simulink model "DeployableEMF"  (R2024a)
settings: Solver=FixedStepAuto  StartTime=0.0  StopTime=0  FixedStep=framePeriod_s  RelTol=1e-3
undefined symbols (not defined in the file): Aircraft, aircraftIC, AircraftModel, Avphi, DiscIntNeverNeededParam, EMF, EnableFF, EnableInputNoise, EnableRCHH, EnableSpeedHold, framePeriod_s, InitCond, Lv, Yv
libraries: simulink x14, simulink_extras x5
(part 2 of 2)

== system DeployableEMF/EMF CLAWS/ACAH EMF1/OnGroundController ==
  cmdsACT : Inport
  Get ACAH Commands1 : Subsystem
      settings: PortSchema="{\"entries\":[{\"content\":{\"sides\":[{\"content\":{\"connectorIds\":[\"In1\"]},\"type\":\"ConnectorPlacement.EquallySpacedRectSide\",\"uuid\":\"7c65b894-e97e-426b-b3a6-5e2b2b7aa780\"},{\"content\":{\"connectorIds\":[\"Out1\"],\"side\":\"RIGHT\"},\"type\":\"ConnectorPlacement.EquallySpacedRectSide\",\"uuid\":\"da5e6856-a2cd-4302-9f49-e9c1cc422564\"},{\"content\":{\"connectorIds\":[\"Out2\"],\"side\":\"TOP\"},\"type\":\"ConnectorPlacement.EquallySpacedRectSide\",\"uuid\":\"a744aea1-4523-47bd-90bf-604bddb972da\"}]},\"type\":\"ConnectorPlacement.EquallySpacedConnector\",\"uuid\":\"254b2f3c-23c2-4cd5-a42e-cd931c0875f5\"}],\"packageUris\":[\"http://schema.mathworks.com/mf0/Connector/R2020b\"],\"version\":\"1.0\"}"
  OL rotor speeds from throttle : Subsystem  Commented=through
  TrimOmegas_OL : Outport
  CmdMoments_Ground : Outport  Port=2
  wires:
  cmdsACT/1 -> Get ACAH Commands1/1(StickInputs)
  Get ACAH Commands1/1(cmdsACAH) -> CmdMoments_Ground/1
  Get ACAH Commands1/2(throttleOmega) -> OL rotor speeds from throttle/1(throttleOmega)
  OL rotor speeds from throttle/1(Omegas_rps) -> TrimOmegas_OL/1

== system DeployableEMF/EMF CLAWS/ACAH EMF1/Rate Saturation ==
  dlat : Inport
  dlon : Inport  Port=2
  dcol : Inport  Port=3
  dped : Inport  Port=4
  Compare To Constant1 : simulink/Logic and Bit Operations/Compare To Constant  relop=<  const=-EMF.MaxCmd.qdot  OutDataTypeStr=boolean
  Compare To Constant2 : simulink/Logic and Bit Operations/Compare To Constant  relop=>  const=EMF.MaxCmd.qdot  OutDataTypeStr=boolean
  Compare To Constant3 : simulink/Logic and Bit Operations/Compare To Constant  relop=<  const=-EMF.MaxCmd.wdot  OutDataTypeStr=boolean
  Compare To Constant4 : simulink/Logic and Bit Operations/Compare To Constant  relop=>  const=EMF.MaxCmd.wdot  OutDataTypeStr=boolean
  Compare To Constant5 : simulink/Logic and Bit Operations/Compare To Constant  relop=<  const=-EMF.MaxCmd.rdot  OutDataTypeStr=boolean
  Compare To Constant6 : simulink/Logic and Bit Operations/Compare To Constant  relop=>  const=EMF.MaxCmd.rdot  OutDataTypeStr=boolean
  Compare To Constant7 : simulink/Logic and Bit Operations/Compare To Constant  relop=<  const=-EMF.MaxCmd.pdot  OutDataTypeStr=boolean
  Compare To Constant8 : simulink/Logic and Bit Operations/Compare To Constant  relop=>  const=EMF.MaxCmd.pdot  OutDataTypeStr=boolean
  Logical Operator{1..4} (4 alike) : Logic  Operator=OR  AllPortsSameDT=off  OutDataTypeStr=boolean
  Mux : Mux
  Saturation : Saturate  UpperLimit=EMF.MaxCmd.pdot  LowerLimit=-EMF.MaxCmd.pdot
  Saturation1 : Saturate  UpperLimit=EMF.MaxCmd.qdot  LowerLimit=-EMF.MaxCmd.qdot
  Saturation2 : Saturate  UpperLimit=EMF.MaxCmd.wdot  LowerLimit=-EMF.MaxCmd.wdot
  Saturation3 : Saturate  UpperLimit=EMF.MaxCmd.rdot  LowerLimit=-EMF.MaxCmd.rdot
  dcol sat : Outport
  dlat sat : Outport  Port=2
  dlon sat : Outport  Port=3
  dped sat : Outport  Port=4
  Flag : Outport  Port=5
  wires:
  Saturation3/1 -> dped sat/1
  Saturation1/1 -> dlon sat/1
  Saturation/1 -> dlat sat/1
  dlat/1 -> Compare To Constant8/1, Compare To Constant7/1, Saturation/1
  Saturation2/1 -> dcol sat/1
  Compare To Constant7/1 -> Logical Operator4/2
  Compare To Constant8/1 -> Logical Operator4/1
  Logical Operator4/1 -> Mux/1
  Logical Operator1/1 -> Mux/2
  Compare To Constant2/1 -> Logical Operator1/1
  Compare To Constant1/1 -> Logical Operator1/2
  dlon/1 -> Compare To Constant2/1, Compare To Constant1/1, Saturation1/1
  dcol/1 -> Compare To Constant3/1, Compare To Constant4/1, Saturation2/1
  Compare To Constant3/1 -> Logical Operator2/2
  Compare To Constant4/1 -> Logical Operator2/1
  Logical Operator2/1 -> Mux/3
  Logical Operator3/1 -> Mux/4
  Compare To Constant6/1 -> Logical Operator3/1
  Compare To Constant5/1 -> Logical Operator3/2
  dped/1 -> Saturation3/1, Compare To Constant6/1, Compare To Constant5/1
  Mux/1 -> Flag/1

== system DeployableEMF/EMF CLAWS/ACAH EMF1/Remap Rotor Speeds to PWM ==
  Rotor Speeds : Inport
  Band-Limited White Noise : simulink/Sources/Band-Limited White Noise  Cov=[1 1 1 1]*0.05  Ts=0.01  seed=[23341 34452 45563 56674]
  Constant1 : Constant  Value=AircraftModel.MinOmegaLimit
  Constant2 : Constant  Value=AircraftModel.MaxOmegaLimit
  Constant3 : Constant  Value=AircraftModel.MinPWMLimit*ones(1,4)
  Constant4 : Constant  Value=AircraftModel.MaxPWMLimit*ones(4,1)
  Data Type Conversion : DataTypeConversion  OutDataTypeStr=int16  SaturateOnIntegerOverflow=off  RndMeth=Floor
  Gain : Gain  Gain=EnableInputNoise
  Rotor Speed Saturation : Subsystem
  Sum1 : Sum  Inputs=|++
  remap : MATLAB Function  TreatAsAtomicUnit=on
  PWM_int16 : Outport
  tag scope: OmSatFlag=global
  wires:
  Sum1/1 -> Data Type Conversion/1  "PWM_cont"
  Rotor Speed Saturation/2(Saturated Rotor Speeds) -> remap/1(norm_in)
  Band-Limited White Noise/1 -> Gain/1
  Rotor Speed Saturation/1(OmegaSaturationFlags) -> [OmSatFlag]
  Data Type Conversion/1 -> PWM_int16/1  "PWM_int16"
  Constant2/1 -> remap/3(in_max)
  remap/1(raw_out) -> Sum1/1  "PWM_cont"
  Constant4/1 -> remap/5(out_max)
  Gain/1 -> Sum1/2
  Constant1/1 -> remap/2(in_min)
  Constant3/1 -> remap/4(out_min)
  Rotor Speeds/1 -> Rotor Speed Saturation/1(Rotor Speeds)

== system DeployableEMF/EMF CLAWS/ACAH EMF1/Subsystem ==
  StateBus : Inport
  Add : Sum  Inputs=+++
  Bus Selector1 : BusSelector  OutputSignals=u_fdbk_mps,v_fdbk_mps,w_fdbk_mps
  Gain : Gain  Gain=0
  Sqrt : Sqrt
  Square : Math  Operator=square
  Square1 : Math  Operator=square
  Square2 : Math  Operator=square
  fps_to_kts : Gain  Gain=0.592484
  Vabs_kts : Outport
  wires:
  Square1/1 -> Add/2
  Bus Selector1/3 -> Square2/1  "<w_fdbk_mps>"
  StateBus/1 -> Bus Selector1/1
  Add/1 -> Sqrt/1
  Square/1 -> Add/1
  Bus Selector1/1 -> Square/1  "<u_fdbk_mps>"
  Bus Selector1/2 -> Gain/1  "<v_fdbk_mps>"
  Sqrt/1 -> fps_to_kts/1
  Square2/1 -> Add/3
  Gain/1 -> Square1/1
  fps_to_kts/1 -> Vabs_kts/1

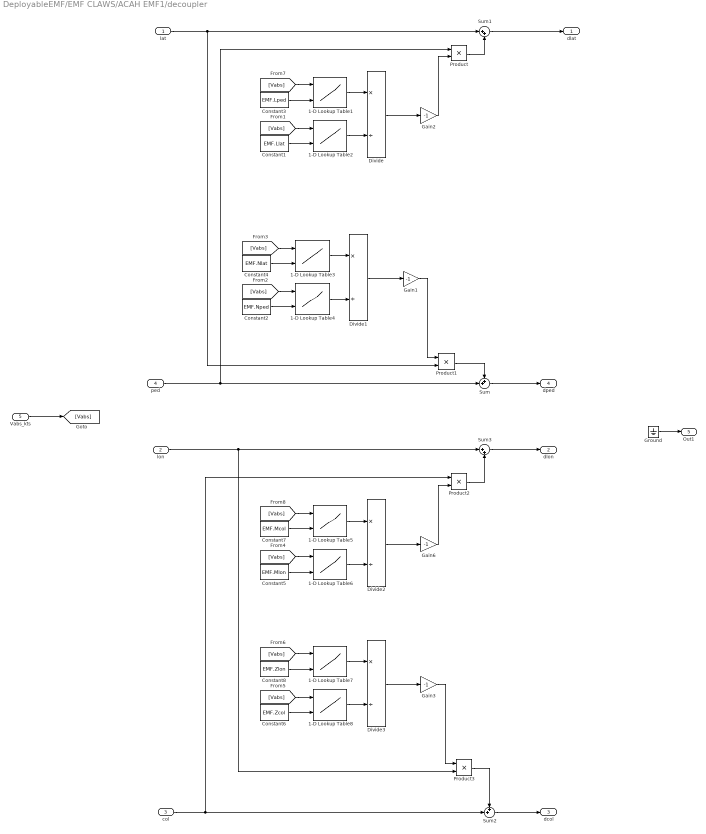
== system DeployableEMF/EMF CLAWS/ACAH EMF1/decoupler ==
  lat : Inport
  lon : Inport  Port=2
  col : Inport  Port=3
  ped : Inport  Port=4
  Vabs_kts : Inport  Port=5
  1-D Lookup Table{1..8} (8 alike) : Lookup_n-D  NumberOfTableDimensions=1  BreakpointsForDimension1=EMF.VTAB  BeginIndexSearchUsingPreviousIndexResult=on  TableSource=Input port  Table=tanh([-5:5])  ExtrapMethod=Clip  InternalRulePriority=Speed  RndMeth=Simplest
      settings: InputPortMap=u0,p221
  Constant1 : Constant  Value=EMF.Llat
  Constant2 : Constant  Value=EMF.Nped
  Constant3 : Constant  Value=EMF.Lped
  Constant4 : Constant  Value=EMF.Nlat
  Constant5 : Constant  Value=EMF.Mlon
  Constant6 : Constant  Value=EMF.Zcol
  Constant7 : Constant  Value=EMF.Mcol
  Constant8 : Constant  Value=EMF.Zlon
  Divide{,1..3} (4 alike) : Product  Inputs=*/
  Gain{1..3,6} (4 alike) : Gain  Gain=-1
  Ground : Ground
  Product{,1..3} (4 alike) : Product
  Sum : Sum  Inputs=++|
  Sum1 : Sum  Inputs=|++
  Sum2 : Sum  Inputs=++|
  Sum3 : Sum  Inputs=|++
  dlat : Outport
  dlon : Outport  Port=2
  dcol : Outport  Port=3
  dped : Outport  Port=4
  Out1 : Outport  Port=5
  wires:
  Vabs_kts/1 -> [Vabs]
  Product3/1 -> Sum2/1
  Product2/1 -> Sum3/2
  Constant7/1 -> 1-D Lookup Table5/2
  [Vabs] -> 1-D Lookup Table5/1
  [Vabs] -> 1-D Lookup Table6/1
  Constant5/1 -> 1-D Lookup Table6/2
  1-D Lookup Table6/1 -> Divide2/2
  1-D Lookup Table5/1 -> Divide2/1
  Divide2/1 -> Gain6/1
  Gain6/1 -> Product2/2
  Gain3/1 -> Product3/1
  Divide3/1 -> Gain3/1
  1-D Lookup Table7/1 -> Divide3/1
  1-D Lookup Table8/1 -> Divide3/2
  Constant6/1 -> 1-D Lookup Table8/2
  [Vabs] -> 1-D Lookup Table8/1
  [Vabs] -> 1-D Lookup Table7/1
  Constant8/1 -> 1-D Lookup Table7/2
  Product1/1 -> Sum/1
  Constant4/1 -> 1-D Lookup Table3/2
  [Vabs] -> 1-D Lookup Table3/1
  [Vabs] -> 1-D Lookup Table4/1
  Constant2/1 -> 1-D Lookup Table4/2
  1-D Lookup Table4/1 -> Divide1/2
  1-D Lookup Table3/1 -> Divide1/1
  Divide1/1 -> Gain1/1
  Gain1/1 -> Product1/1
  Gain2/1 -> Product/2
  Product/1 -> Sum1/2
  Divide/1 -> Gain2/1
  1-D Lookup Table1/1 -> Divide/1
  1-D Lookup Table2/1 -> Divide/2
  Constant1/1 -> 1-D Lookup Table2/2
  [Vabs] -> 1-D Lookup Table2/1
  [Vabs] -> 1-D Lookup Table1/1
  Constant3/1 -> 1-D Lookup Table1/2
  Sum3/1 -> dlon/1
  Sum2/1 -> dcol/1
  Sum1/1 -> dlat/1
  ped/1 -> Sum/2, Product/1
  lat/1 -> Sum1/1, Product1/2
  Sum/1 -> dped/1
  col/1 -> Product2/1, Sum2/2
  lon/1 -> Product3/2, Sum3/1
  Ground/1 -> Out1/1

== system DeployableEMF/EMF CLAWS/ACAH EMF1/Inner Loop - ACAH/A-channel Delay ==
  p_ideal : Inport
  phi_ideal : Inport  Port=2
  Constant : Constant  Value=EMF.tauf
  Demux : Demux  Outputs=2
  Divide : Product  Inputs=*/
  Integrator : Integrator
  Mux : Mux  Inputs=2
  Sum : Sum  Inputs=|+-
  p_ideal_delayed : Outport
  phi_ideal_delayed : Outport  Port=2
  wires:
  Demux/2 -> phi_ideal_delayed/1
  Demux/1 -> p_ideal_delayed/1
  phi_ideal/1 -> Mux/2
  p_ideal/1 -> Mux/1
  Mux/1 -> Sum/1
  Constant/1 -> Divide/2
  Divide/1 -> Integrator/1
  Sum/1 -> Divide/1
  Integrator/1 -> Demux/1, Sum/2

== system DeployableEMF/EMF CLAWS/ACAH EMF1/Inner Loop - ACAH/B-channel Delay ==
  q_ideal : Inport
  tht_ideal : Inport  Port=2
  Constant : Constant  Value=EMF.tauf
  Demux : Demux  Outputs=2
  Divide : Product  Inputs=*/
  Integrator : Integrator
  Mux : Mux  Inputs=2
  Sum : Sum  Inputs=|+-
  q_ideal_delayed : Outport
  tht_ideal_delayed : Outport  Port=2
  wires:
  Demux/2 -> tht_ideal_delayed/1
  Demux/1 -> q_ideal_delayed/1
  tht_ideal/1 -> Mux/2
  q_ideal/1 -> Mux/1
  Mux/1 -> Sum/1
  Constant/1 -> Divide/2
  Divide/1 -> Integrator/1
  Sum/1 -> Divide/1
  Integrator/1 -> Demux/1, Sum/2

== system DeployableEMF/EMF CLAWS/ACAH EMF1/Inner Loop - ACAH/C-channel Delay ==
  w_ideal : Inport
  Constant : Constant  Value=EMF.tauf
  Divide : Product  Inputs=*/
  Integrator : Integrator
  Sum : Sum  Inputs=|+-
  w_ideal_delay : Outport
  wires:
  w_ideal/1 -> Sum/1
  Constant/1 -> Divide/2
  Divide/1 -> Integrator/1
  Sum/1 -> Divide/1
  Integrator/1 -> w_ideal_delay/1, Sum/2

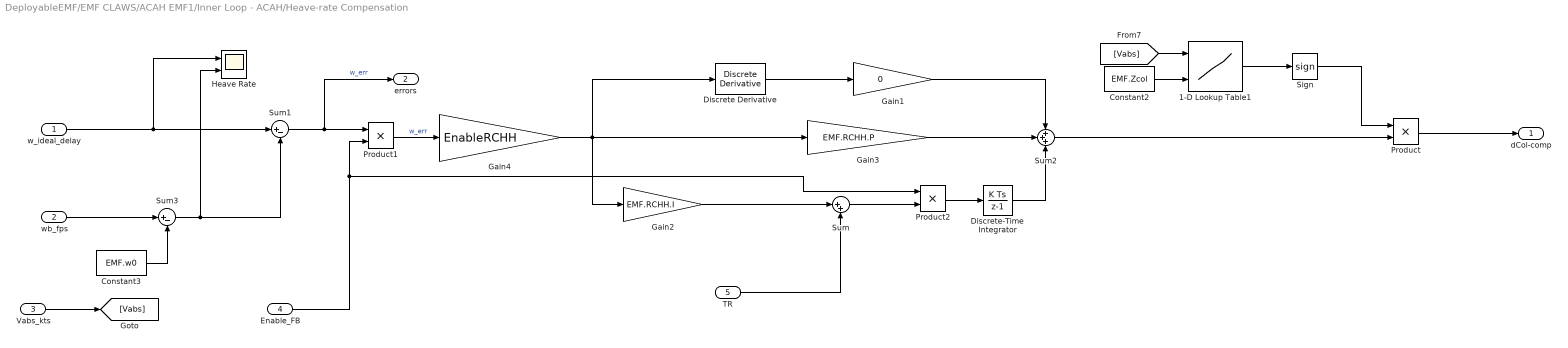
== system DeployableEMF/EMF CLAWS/ACAH EMF1/Inner Loop - ACAH/Heave-rate Compensation ==
  w_ideal_delay : Inport
  wb_fps : Inport  Port=2
  Vabs_kts : Inport  Port=3
  Enable_FB : Inport  Port=4
  TR : Inport  Port=5
  1-D Lookup Table1 : Lookup_n-D  NumberOfTableDimensions=1  BreakpointsForDimension1=EMF.VTAB  BeginIndexSearchUsingPreviousIndexResult=on  TableSource=Input port  Table=tanh([-5:5])  ExtrapMethod=Clip  InternalRulePriority=Speed  RndMeth=Simplest
      settings: InputPortMap=u0,p221
  Constant2 : Constant  Value=EMF.Zcol
  Constant3 : Constant  Value=EMF.w0
  Discrete Derivative : simulink/Discrete/Discrete Derivative  gainval=1.0  ICPrevScaledInput=0.0  OutMin=[]  OutMax=[]  OutDataType=fixdt(1, 16)  OutScaling=2^-10  DoSatur=off
  Discrete-Time Integrator : DiscreteIntegrator  SampleTime=-1  ICPrevOutput=DiscIntNeverNeededParam  ICPrevScaledInput=DiscIntNeverNeededParam
  Gain1 : Gain  Gain=0
  Gain2 : Gain  Gain=EMF.RCHH.I
  Gain3 : Gain  Gain=EMF.RCHH.P
  Gain4 : Gain  Gain=EnableRCHH
  Heave Rate : Scope  NumInputPorts=2
  Product : Product
  Product1 : Product
  Product2 : Product
  Sign : Signum
  Sum : Sum  Inputs=|++
  Sum1 : Sum  Inputs=|+-
  Sum2 : Sum  Inputs=+++
  Sum3 : Sum  Inputs=|+-
  dCol-comp : Outport
  errors : Outport  Port=2
  wires:
  Gain3/1 -> Sum2/2
  Sum/1 -> Product2/2
  wb_fps/1 -> Sum3/1
  Sign/1 -> Product/1
  1-D Lookup Table1/1 -> Sign/1
  Product/1 -> dCol-comp/1
  Discrete Derivative/1 -> Gain1/1
  Product1/1 -> Gain4/1  "w_err"
  Sum2/1 -> Product/2
  Gain1/1 -> Sum2/1
  w_ideal_delay/1 -> Heave Rate/1, Sum1/1
  [Vabs] -> 1-D Lookup Table1/1
  Constant2/1 -> 1-D Lookup Table1/2
  Vabs_kts/1 -> [Vabs]
  Sum3/1 -> Heave Rate/2, Sum1/2
  Constant3/1 -> Sum3/2
  Sum1/1 -> errors/1, Product1/1  "w_err"
  Enable_FB/1 -> Product2/1, Product1/2
  Discrete-Time Integrator/1 -> Sum2/3
  Product2/1 -> Discrete-Time Integrator/1
  Gain2/1 -> Sum/1
  TR/1 -> Sum/2
  Gain4/1 -> Discrete Derivative/1, Gain3/1, Gain2/1

== system DeployableEMF/EMF CLAWS/ACAH EMF1/Inner Loop - ACAH/P-channel Delay ==
  r_ideal : Inport
  Constant : Constant  Value=EMF.tauf
  Divide : Product  Inputs=*/
  Integrator : Integrator
  Sum : Sum  Inputs=|+-
  r_ideal_delay : Outport
  wires:
  Divide/1 -> Integrator/1
  r_ideal/1 -> Sum/1
  Integrator/1 -> Sum/2, r_ideal_delay/1
  Constant/1 -> Divide/2
  Sum/1 -> Divide/1

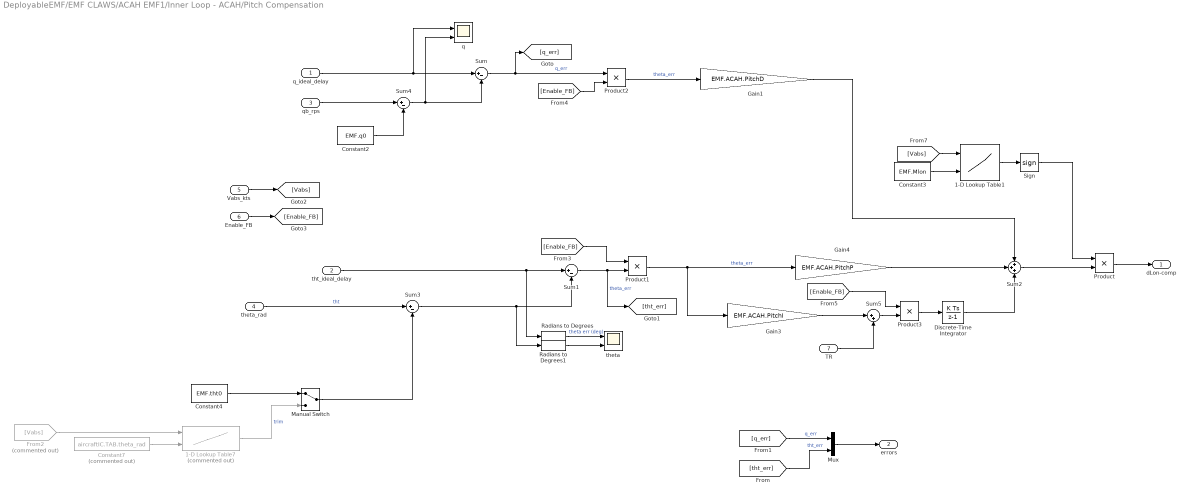
== system DeployableEMF/EMF CLAWS/ACAH EMF1/Inner Loop - ACAH/Pitch Compensation ==
  q_ideal_delay : Inport
  tht_ideal_delay : Inport  Port=2
  qb_rps : Inport  Port=3
  theta_rad : Inport  Port=4
  Vabs_kts : Inport  Port=5
  Enable_FB : Inport  Port=6
  TR : Inport  Port=7
  1-D Lookup Table1 : Lookup_n-D  NumberOfTableDimensions=1  BreakpointsForDimension1=EMF.VTAB  BeginIndexSearchUsingPreviousIndexResult=on  TableSource=Input port  Table=tanh([-5:5])  ExtrapMethod=Clip  InternalRulePriority=Speed  RndMeth=Simplest
      settings: InputPortMap=u0,p221
  1-D Lookup Table7 : Lookup_n-D  Commented=on  NumberOfTableDimensions=1  BreakpointsForDimension1=EMF.VTAB  BeginIndexSearchUsingPreviousIndexResult=on  TableSource=Input port  Table=tanh([-5:5])  ExtrapMethod=Clip  InternalRulePriority=Speed  RndMeth=Simplest
      settings: InputPortMap=u0,p221
  Constant2 : Constant  Value=EMF.q0
  Constant3 : Constant  Value=EMF.Mlon
  Constant4 : Constant  Value=EMF.tht0
  Constant7 : Constant  Commented=on  Value=aircraftIC.TAB.theta_rad
  Discrete-Time Integrator : DiscreteIntegrator  SampleTime=-1  ICPrevOutput=DiscIntNeverNeededParam  ICPrevScaledInput=DiscIntNeverNeededParam
  From2 : From  Commented=on  GotoTag=Vabs
  Gain1 : Gain  Gain=EMF.ACAH.PitchD
  Gain3 : Gain  Gain=EMF.ACAH.PitchI
  Gain4 : Gain  Gain=EMF.ACAH.PitchP
  Manual Switch : ManualSwitch
  Mux : Mux  Inputs=2
  Product{,1..3} (4 alike) : Product
  Radians to Degrees : simulink_extras/Transformations/Radians to Degrees
  Radians to Degrees1 : simulink_extras/Transformations/Radians to Degrees
  Sign : Signum
  Sum{,1,3..4} (4 alike) : Sum  Inputs=|+-
  Sum2 : Sum  Inputs=+++
  Sum5 : Sum  Inputs=|++
  q : Scope  NumInputPorts=2
  theta : Scope  NumInputPorts=2
  dLon-comp : Outport
  errors : Outport  Port=2
  wires:
  Gain4/1 -> Sum2/2
  Sign/1 -> Product/1
  Product/1 -> dLon-comp/1
  Gain1/1 -> Sum2/1
  [q_err] -> Mux/1  "q_err"
  Mux/1 -> errors/1
  [tht_err] -> Mux/2  "tht_err"
  Sum/1 -> Product2/1, [q_err]  "q_err"
  Product1/1 -> Gain3/1, Gain4/1  "theta_err"
  q_ideal_delay/1 -> Sum/1, q/1
  qb_rps/1 -> Sum4/1
  Sum4/1 -> Sum/2, q/2
  Constant2/1 -> Sum4/2
  [Vabs] -> 1-D Lookup Table1/1
  Constant3/1 -> 1-D Lookup Table1/2
  1-D Lookup Table1/1 -> Sign/1
  Vabs_kts/1 -> [Vabs]
  Radians to Degrees/1 -> theta/1  "theta err (deg)"
  Radians to Degrees1/1 -> theta/2
  Constant7/1 -> 1-D Lookup Table7/2
  Constant4/1 -> Manual Switch/1
  Sum3/1 -> Sum1/2, Radians to Degrees1/1
  From2/1 -> 1-D Lookup Table7/1
  theta_rad/1 -> Sum3/1  "tht"
  1-D Lookup Table7/1 -> Manual Switch/2  "trim"
  Sum5/1 -> Product3/2
  tht_ideal_delay/1 -> Sum1/1, Radians to Degrees/1
  Sum2/1 -> Product/2
  Manual Switch/1 -> Sum3/2
  Sum1/1 -> [tht_err], Product1/2  "theta_err"
  Enable_FB/1 -> [Enable_FB]
  [Enable_FB] -> Product1/1
  Product2/1 -> Gain1/1  "theta_err"
  [Enable_FB] -> Product2/2
  Discrete-Time Integrator/1 -> Sum2/3
  Product3/1 -> Discrete-Time Integrator/1
  [Enable_FB] -> Product3/1
  Gain3/1 -> Sum5/1
  TR/1 -> Sum5/2

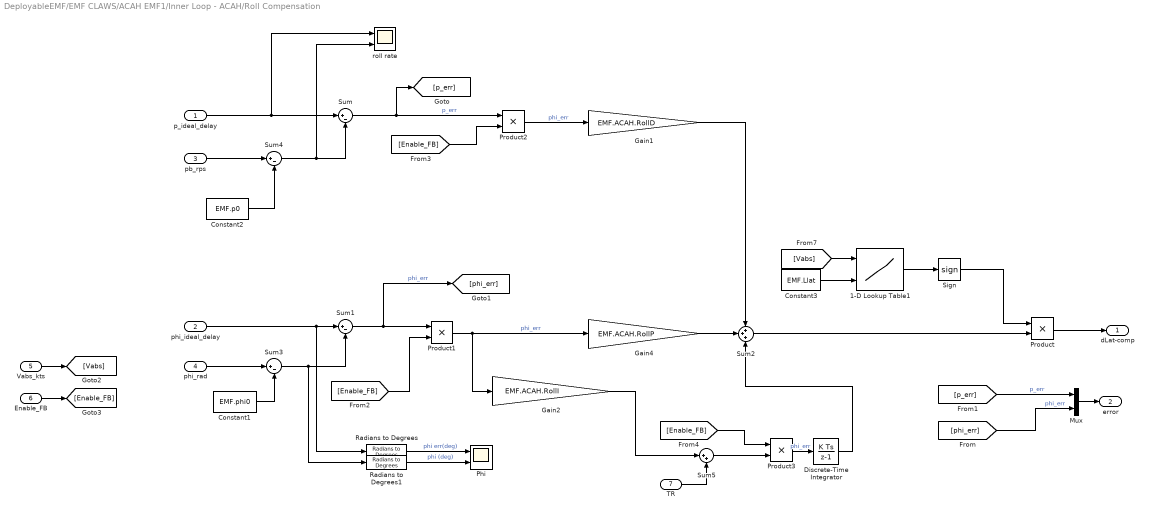
== system DeployableEMF/EMF CLAWS/ACAH EMF1/Inner Loop - ACAH/Roll Compensation ==
  p_ideal_delay : Inport
  phi_ideal_delay : Inport  Port=2
  pb_rps : Inport  Port=3
  phi_rad : Inport  Port=4
  Vabs_kts : Inport  Port=5
  Enable_FB : Inport  Port=6
  TR : Inport  Port=7
  1-D Lookup Table1 : Lookup_n-D  NumberOfTableDimensions=1  BreakpointsForDimension1=EMF.VTAB  BeginIndexSearchUsingPreviousIndexResult=on  TableSource=Input port  Table=tanh([-5:5])  ExtrapMethod=Clip  InternalRulePriority=Speed  RndMeth=Simplest
      settings: InputPortMap=u0,p221
  Constant1 : Constant  Value=EMF.phi0
  Constant2 : Constant  Value=EMF.p0
  Constant3 : Constant  Value=EMF.Llat
  Discrete-Time Integrator : DiscreteIntegrator  SampleTime=-1  ICPrevOutput=DiscIntNeverNeededParam  ICPrevScaledInput=DiscIntNeverNeededParam
  Gain1 : Gain  Gain=EMF.ACAH.RollD
  Gain2 : Gain  Gain=EMF.ACAH.RollI
  Gain4 : Gain  Gain=EMF.ACAH.RollP
  Mux : Mux  Inputs=2
  Phi : Scope  NumInputPorts=2
  Product{,1..3} (4 alike) : Product
  Radians to Degrees : simulink_extras/Transformations/Radians to Degrees
  Radians to Degrees1 : simulink_extras/Transformations/Radians to Degrees
  Sign : Signum
  Sum{,1,3..4} (4 alike) : Sum  Inputs=|+-
  Sum2 : Sum  Inputs=+++
  Sum5 : Sum  Inputs=|++
  roll rate : Scope  NumInputPorts=2
  dLat-comp : Outport
  error : Outport  Port=2
  wires:
  Gain4/1 -> Sum2/2
  Sum2/1 -> Product/2
  Sign/1 -> Product/1
  Product/1 -> dLat-comp/1
  [phi_err] -> Mux/2  "phi_err"
  phi_ideal_delay/1 -> Sum1/1, Radians to Degrees/1
  phi_rad/1 -> Sum3/1
  Sum/1 -> [p_err], Product2/1  "p_err"
  Gain1/1 -> Sum2/1
  Product1/1 -> Gain2/1, Gain4/1  "phi_err"
  p_ideal_delay/1 -> Sum/1, roll rate/1
  Sum3/1 -> Radians to Degrees1/1, Sum1/2
  Constant1/1 -> Sum3/2
  Sum4/1 -> Sum/2, roll rate/2
  Constant2/1 -> Sum4/2
  pb_rps/1 -> Sum4/1
  [Vabs] -> 1-D Lookup Table1/1
  Constant3/1 -> 1-D Lookup Table1/2
  Vabs_kts/1 -> [Vabs]
  1-D Lookup Table1/1 -> Sign/1
  Sum5/1 -> Product3/2
  Radians to Degrees/1 -> Phi/1  "phi err(deg)"
  Radians to Degrees1/1 -> Phi/2  "phi (deg)"
  Enable_FB/1 -> [Enable_FB]
  Sum1/1 -> [phi_err], Product1/1  "phi_err"
  [Enable_FB] -> Product1/2
  Product2/1 -> Gain1/1  "phi_err"
  [Enable_FB] -> Product2/2
  Discrete-Time Integrator/1 -> Sum2/3
  Product3/1 -> Discrete-Time Integrator/1  "phi_err"
  [Enable_FB] -> Product3/1
  Gain2/1 -> Sum5/1
  TR/1 -> Sum5/2
  Mux/1 -> error/1
  [p_err] -> Mux/1  "p_err"

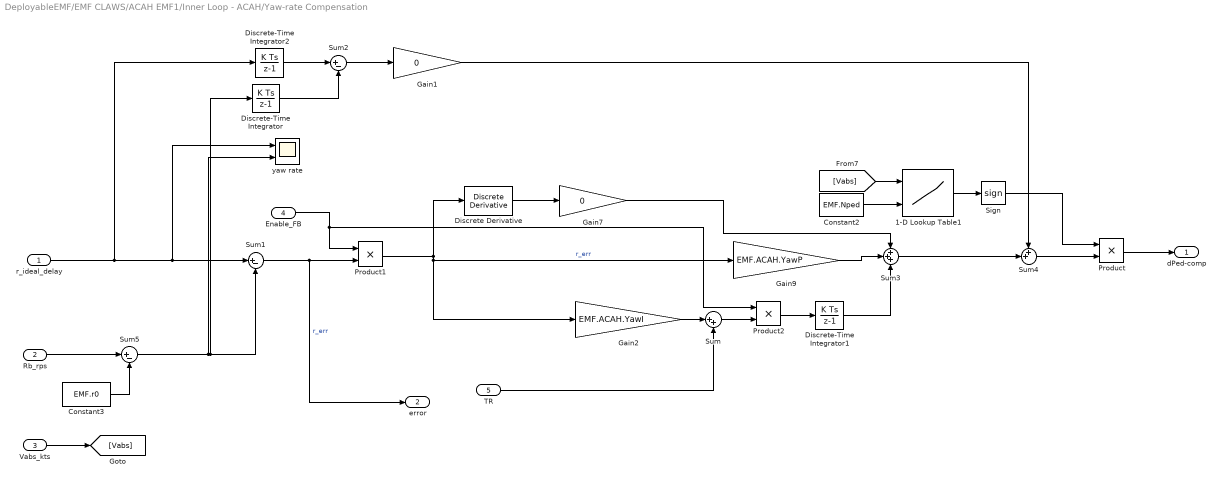
== system DeployableEMF/EMF CLAWS/ACAH EMF1/Inner Loop - ACAH/Yaw-rate Compensation ==
  r_ideal_delay : Inport
  Rb_rps : Inport  Port=2
  Vabs_kts : Inport  Port=3
  Enable_FB : Inport  Port=4
  TR : Inport  Port=5
  1-D Lookup Table1 : Lookup_n-D  NumberOfTableDimensions=1  BreakpointsForDimension1=EMF.VTAB  BeginIndexSearchUsingPreviousIndexResult=on  TableSource=Input port  Table=tanh([-5:5])  ExtrapMethod=Clip  InternalRulePriority=Speed  RndMeth=Simplest
      settings: InputPortMap=u0,p221
  Constant2 : Constant  Value=EMF.Nped
  Constant3 : Constant  Value=EMF.r0
  Discrete Derivative : simulink/Discrete/Discrete Derivative  gainval=1.0  ICPrevScaledInput=0.0  OutMin=[]  OutMax=[]  OutDataType=fixdt(1, 16)  OutScaling=2^-10  DoSatur=off
  Discrete-Time Integrator : DiscreteIntegrator  SampleTime=-1  ICPrevOutput=DiscIntNeverNeededParam  ICPrevScaledInput=DiscIntNeverNeededParam
  Discrete-Time Integrator1 : DiscreteIntegrator  SampleTime=-1  ICPrevOutput=DiscIntNeverNeededParam  ICPrevScaledInput=DiscIntNeverNeededParam
  Discrete-Time Integrator2 : DiscreteIntegrator  SampleTime=-1  ICPrevOutput=DiscIntNeverNeededParam  ICPrevScaledInput=DiscIntNeverNeededParam
  Gain1 : Gain  Gain=0
  Gain2 : Gain  Gain=EMF.ACAH.YawI
  Gain7 : Gain  Gain=0
  Gain9 : Gain  Gain=EMF.ACAH.YawP
  Product : Product
  Product1 : Product
  Product2 : Product
  Sign : Signum
  Sum : Sum  Inputs=|++
  Sum1 : Sum  Inputs=|+-
  Sum2 : Sum  Inputs=|+-
  Sum3 : Sum  Inputs=+++
  Sum4 : Sum  Inputs=++|
  Sum5 : Sum  Inputs=|+-
  yaw rate : Scope  NumInputPorts=2
  dPed-comp : Outport
  error : Outport  Port=2
  wires:
  Product1/1 -> Discrete Derivative/1, Gain2/1, Gain9/1  "r_err"
  Discrete Derivative/1 -> Gain7/1
  Gain7/1 -> Sum3/1
  Gain9/1 -> Sum3/2
  Sum/1 -> Product2/2
  Sign/1 -> Product/1
  Product/1 -> dPed-comp/1
  1-D Lookup Table1/1 -> Sign/1
  Rb_rps/1 -> Sum5/1
  r_ideal_delay/1 -> Discrete-Time Integrator2/1, Sum1/1, yaw rate/1
  Discrete-Time Integrator2/1 -> Sum2/1
  Discrete-Time Integrator/1 -> Sum2/2
  Sum2/1 -> Gain1/1
  Sum3/1 -> Sum4/2
  Sum4/1 -> Product/2
  Gain1/1 -> Sum4/1
  [Vabs] -> 1-D Lookup Table1/1
  Constant2/1 -> 1-D Lookup Table1/2
  Vabs_kts/1 -> [Vabs]
  Sum5/1 -> Discrete-Time Integrator/1, Sum1/2, yaw rate/2
  Constant3/1 -> Sum5/2
  Enable_FB/1 -> Product2/1, Product1/1
  Sum1/1 -> error/1, Product1/2  "r_err"
  Discrete-Time Integrator1/1 -> Sum3/3
  Product2/1 -> Discrete-Time Integrator1/1
  Gain2/1 -> Sum/1
  TR/1 -> Sum/2

== system DeployableEMF/EMF CLAWS/ACAH EMF1/Inner Loop - ACAH/[Heave] Cmd Filter // Inv Model ==
  note: Inverse Model
  note: Command Filter
  w_cmd (ft/s) : Inport
  Vabs_kts : Inport  Port=2
  1-D Lookup Table : Lookup_n-D  NumberOfTableDimensions=1  BreakpointsForDimension1=EMF.VTAB  BeginIndexSearchUsingPreviousIndexResult=on  TableSource=Input port  Table=tanh([-5:5])  ExtrapMethod=Clip  InternalRulePriority=Speed  OutDataTypeStr=single  RndMeth=Simplest
      settings: InputPortMap=u0,p221
  1-D Lookup Table1 : Lookup_n-D  NumberOfTableDimensions=1  BreakpointsForDimension1=EMF.VTAB  BeginIndexSearchUsingPreviousIndexResult=on  TableSource=Input port  Table=tanh([-5:5])  ExtrapMethod=Clip  InternalRulePriority=Speed  OutDataTypeStr=single  RndMeth=Simplest
      settings: InputPortMap=u0,p221
  Bus Creator : BusCreator  Inputs=2
  Constant : Constant  Value=EMF.wTau  OutDataTypeStr=single
  Constant1 : Constant  Value=EMF.Zw  OutDataTypeStr=single
  Constant3 : Constant  Value=EMF.Zcol  OutDataTypeStr=single
  Delay : Delay  DelayLength=EMF.HeaveDelay/framePeriod_s
  Delay1 : Delay  DelayLength=EMF.HeaveDelay/framePeriod_s
  Discrete-Time Integrator : DiscreteIntegrator  SampleTime=-1  OutDataTypeStr=single  ICPrevOutput=DiscIntNeverNeededParam  ICPrevScaledInput=DiscIntNeverNeededParam
  Divide : Product  Inputs=*/  OutDataTypeStr=single
  Divide1 : Product  Inputs=*/  OutDataTypeStr=single
  Product3 : Product
  Sum : Sum  Inputs=|+-
  Sum2 : Sum  Inputs=|+-
  col_ff : Outport
  w_ideal : Outport  Port=2
  cmdFilValues : Outport  Port=3
  wires:
  [wdot_ideal] -> Delay/1  "wdot_ideal"
  [w_ideal] -> Delay1/1  "Vz_ideal"
  Bus Creator/1 -> cmdFilValues/1
  Divide/1 -> Discrete-Time Integrator/1, Sum2/1, [wdot_ideal]  "wdot_ideal"
  Discrete-Time Integrator/1 -> w_ideal/1, [w_ideal], Product3/2, Sum/2  "w_ideal"
  Sum/1 -> Divide/1
  w_cmd (ft/s)/1 -> Sum/1
  Sum2/1 -> Divide1/1
  Constant/1 -> Divide/2
  Product3/1 -> Sum2/2
  Divide1/1 -> col_ff/1
  [Vabs] -> 1-D Lookup Table/1
  Constant1/1 -> 1-D Lookup Table/2
  1-D Lookup Table/1 -> Product3/1
  [Vabs] -> 1-D Lookup Table1/1
  Constant3/1 -> 1-D Lookup Table1/2
  1-D Lookup Table1/1 -> Divide1/2
  Vabs_kts/1 -> [Vabs]
  Delay/1 -> Bus Creator/1  "Vzdot_filtered"
  Delay1/1 -> Bus Creator/2  "Vz_filtered"

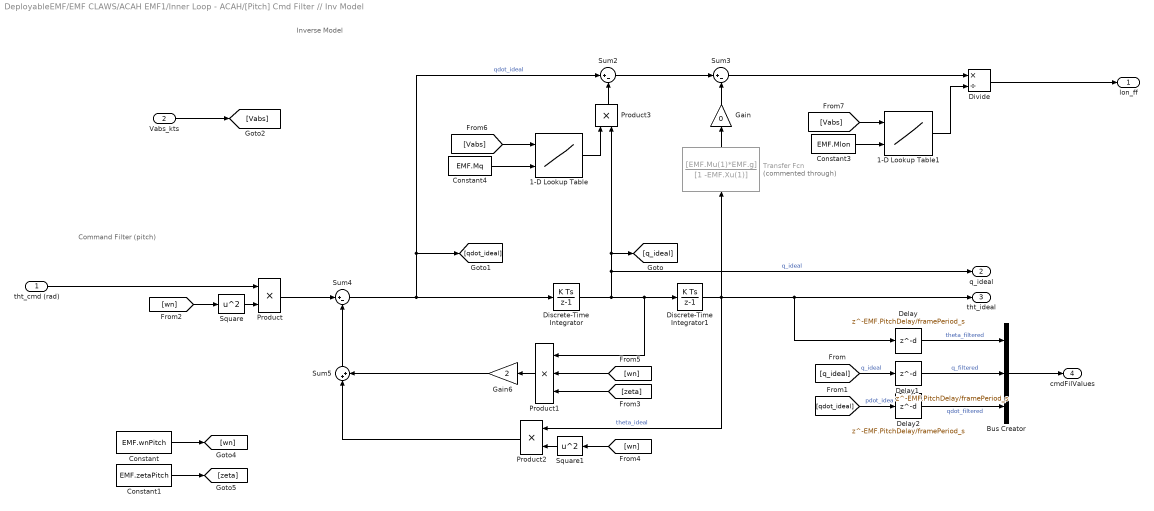
== system DeployableEMF/EMF CLAWS/ACAH EMF1/Inner Loop - ACAH/[Pitch] Cmd Filter // Inv Model ==
  note: Command Filter (pitch)
  note: Inverse Model
  tht_cmd (rad) : Inport
  Vabs_kts : Inport  Port=2
  1-D Lookup Table : Lookup_n-D  NumberOfTableDimensions=1  BreakpointsForDimension1=EMF.VTAB  BeginIndexSearchUsingPreviousIndexResult=on  TableSource=Input port  Table=tanh([-5:5])  ExtrapMethod=Clip  InternalRulePriority=Speed  RndMeth=Simplest
      settings: InputPortMap=u0,p221
  1-D Lookup Table1 : Lookup_n-D  NumberOfTableDimensions=1  BreakpointsForDimension1=EMF.VTAB  BeginIndexSearchUsingPreviousIndexResult=on  TableSource=Input port  Table=tanh([-5:5])  ExtrapMethod=Clip  InternalRulePriority=Speed  RndMeth=Simplest
      settings: InputPortMap=u0,p221
  Bus Creator : BusCreator  Inputs=3
  Constant : Constant  Value=EMF.wnPitch
  Constant1 : Constant  Value=EMF.zetaPitch
  Constant3 : Constant  Value=EMF.Mlon
  Constant4 : Constant  Value=EMF.Mq
  Delay : Delay  DelayLength=EMF.PitchDelay/framePeriod_s
  Delay1 : Delay  DelayLength=EMF.PitchDelay/framePeriod_s
  Delay2 : Delay  DelayLength=EMF.PitchDelay/framePeriod_s
  Discrete-Time Integrator : DiscreteIntegrator  SampleTime=-1  ICPrevOutput=DiscIntNeverNeededParam  ICPrevScaledInput=DiscIntNeverNeededParam
  Discrete-Time Integrator1 : DiscreteIntegrator  SampleTime=-1  ICPrevOutput=DiscIntNeverNeededParam  ICPrevScaledInput=DiscIntNeverNeededParam
  Divide : Product  Inputs=*/
  Gain : Gain  Gain=0
  Gain6 : Gain  Gain=2
  Product : Product
  Product1 : Product  Inputs=3
  Product2 : Product
  Product3 : Product
  Square : Math  Operator=square
  Square1 : Math  Operator=square
  Sum2 : Sum  Inputs=|+-
  Sum3 : Sum  Inputs=|+-
  Sum4 : Sum  Inputs=|+-
  Sum5 : Sum  Inputs=|++
  Transfer Fcn : TransferFcn  Commented=through  Numerator=[EMF.Mu(1)*EMF.g]  Denominator=[1 -EMF.Xu(1)]
  lon_ff : Outport
  q_ideal : Outport  Port=2
  tht_ideal : Outport  Port=3
  cmdFilValues : Outport  Port=4
  wires:
  [q_ideal] -> Delay1/1  "q_ideal"
  [qdot_ideal] -> Delay2/1  "pdot_idea"
  Bus Creator/1 -> cmdFilValues/1
  Sum2/1 -> Sum3/1
  tht_cmd (rad)/1 -> Product/1
  Transfer Fcn/1 -> Gain/1
  [wn] -> Product1/2
  Product1/1 -> Gain6/1
  [zeta] -> Product1/3
  Constant1/1 -> [zeta]
  Gain6/1 -> Sum5/2
  Product/1 -> Sum4/1
  Constant/1 -> [wn]
  Square1/1 -> Product2/2
  [wn] -> Square1/1
  Square/1 -> Product/2
  Discrete-Time Integrator/1 -> Product3/2, [q_ideal], q_ideal/1, Discrete-Time Integrator1/1, Product1/1  "q_ideal"
  [wn] -> Square/1
  Discrete-Time Integrator1/1 -> Delay/1, tht_ideal/1, Transfer Fcn/1, Product2/1  "theta_ideal"
  Sum4/1 -> Discrete-Time Integrator/1, [qdot_ideal], Sum2/1  "qdot_ideal"
  Sum5/1 -> Sum4/2
  Product2/1 -> Sum5/1
  1-D Lookup Table/1 -> Product3/1
  Product3/1 -> Sum2/2
  Sum3/1 -> Divide/1
  Divide/1 -> lon_ff/1
  Gain/1 -> Sum3/2
  [Vabs] -> 1-D Lookup Table/1
  Constant4/1 -> 1-D Lookup Table/2
  Constant3/1 -> 1-D Lookup Table1/2
  1-D Lookup Table1/1 -> Divide/2
  [Vabs] -> 1-D Lookup Table1/1
  Vabs_kts/1 -> [Vabs]
  Delay/1 -> Bus Creator/1  "theta_filtered"
  Delay1/1 -> Bus Creator/2  "q_filtered"
  Delay2/1 -> Bus Creator/3  "qdot_filtered"

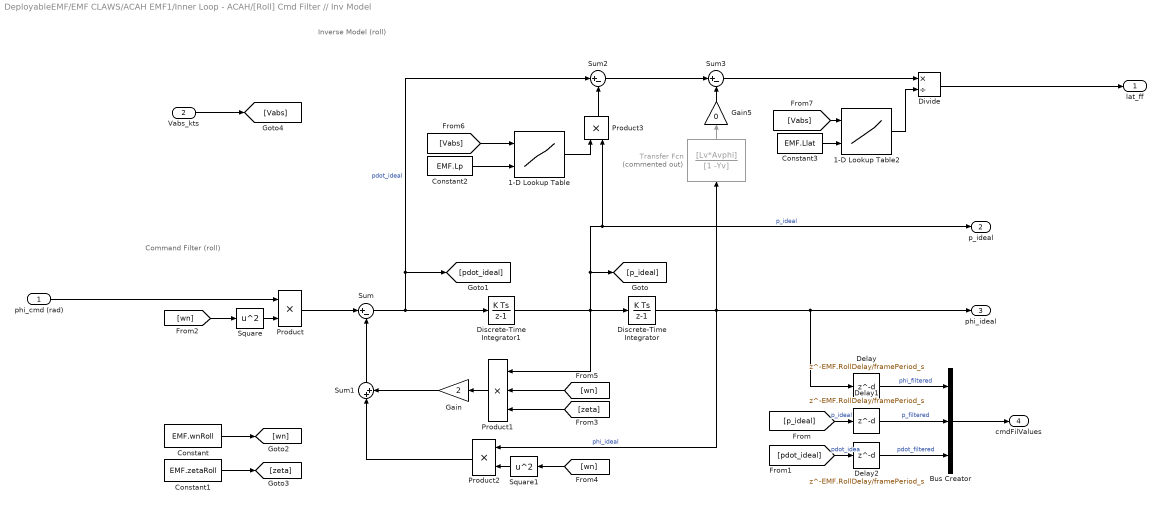
== system DeployableEMF/EMF CLAWS/ACAH EMF1/Inner Loop - ACAH/[Roll] Cmd Filter // Inv Model ==
  note: Command Filter (roll)
  note: Inverse Model (roll)
  phi_cmd (rad) : Inport
  Vabs_kts : Inport  Port=2
  1-D Lookup Table : Lookup_n-D  NumberOfTableDimensions=1  BreakpointsForDimension1=EMF.VTAB  BeginIndexSearchUsingPreviousIndexResult=on  TableSource=Input port  Table=tanh([-5:5])  ExtrapMethod=Clip  InternalRulePriority=Speed  RndMeth=Simplest
      settings: InputPortMap=u0,p221
  1-D Lookup Table2 : Lookup_n-D  NumberOfTableDimensions=1  BreakpointsForDimension1=EMF.VTAB  BeginIndexSearchUsingPreviousIndexResult=on  TableSource=Input port  Table=tanh([-5:5])  ExtrapMethod=Clip  InternalRulePriority=Speed  RndMeth=Simplest
      settings: InputPortMap=u0,p221
  Bus Creator : BusCreator  Inputs=3
  Constant : Constant  Value=EMF.wnRoll
  Constant1 : Constant  Value=EMF.zetaRoll
  Constant2 : Constant  Value=EMF.Lp
  Constant3 : Constant  Value=EMF.Llat
  Delay : Delay  DelayLength=EMF.RollDelay/framePeriod_s
  Delay1 : Delay  DelayLength=EMF.RollDelay/framePeriod_s
  Delay2 : Delay  DelayLength=EMF.RollDelay/framePeriod_s
  Discrete-Time Integrator : DiscreteIntegrator  SampleTime=-1  ICPrevOutput=DiscIntNeverNeededParam  ICPrevScaledInput=DiscIntNeverNeededParam
  Discrete-Time Integrator1 : DiscreteIntegrator  SampleTime=-1  ICPrevOutput=DiscIntNeverNeededParam  ICPrevScaledInput=DiscIntNeverNeededParam
  Divide : Product  Inputs=*/
  Gain : Gain  Gain=2
  Gain5 : Gain  Gain=0
  Product : Product
  Product1 : Product  Inputs=3
  Product2 : Product
  Product3 : Product
  Square : Math  Operator=square
  Square1 : Math  Operator=square
  Sum : Sum  Inputs=|+-
  Sum1 : Sum  Inputs=|++
  Sum2 : Sum  Inputs=|+-
  Sum3 : Sum  Inputs=|+-
  Transfer Fcn : TransferFcn  Commented=on  Numerator=[Lv*Avphi]  Denominator=[1 -Yv]
  lat_ff : Outport
  p_ideal : Outport  Port=2
  phi_ideal : Outport  Port=3
  cmdFilValues : Outport  Port=4
  wires:
  Transfer Fcn/1 -> Gain5/1
  Sum2/1 -> Sum3/1
  Sum3/1 -> Divide/1
  Bus Creator/1 -> cmdFilValues/1
  [pdot_ideal] -> Delay2/1  "pdot_idea"
  [p_ideal] -> Delay1/1  "p_ideal"
  Product3/1 -> Sum2/2
  Divide/1 -> lat_ff/1
  Product2/1 -> Sum1/1
  Sum1/1 -> Sum/2
  Product/1 -> Sum/1
  Sum/1 -> Discrete-Time Integrator1/1, [pdot_ideal], Sum2/1  "pdot_ideal"
  Gain/1 -> Sum1/2
  Discrete-Time Integrator/1 -> Product2/1, Transfer Fcn/1, Delay/1, phi_ideal/1  "phi_ideal"
  Discrete-Time Integrator1/1 -> Discrete-Time Integrator/1, Product1/1, [p_ideal], Product3/2, p_ideal/1  "p_ideal"
  phi_cmd (rad)/1 -> Product/1
  Gain5/1 -> Sum3/2
  Square/1 -> Product/2
  Constant/1 -> [wn]
  [wn] -> Square/1
  Constant1/1 -> [zeta]
  [wn] -> Square1/1
  Square1/1 -> Product2/2
  [zeta] -> Product1/3
  [wn] -> Product1/2
  Product1/1 -> Gain/1
  Constant2/1 -> 1-D Lookup Table/2
  1-D Lookup Table/1 -> Product3/1
  Constant3/1 -> 1-D Lookup Table2/2
  1-D Lookup Table2/1 -> Divide/2
  Vabs_kts/1 -> [Vabs]
  [Vabs] -> 1-D Lookup Table/1
  [Vabs] -> 1-D Lookup Table2/1
  Delay/1 -> Bus Creator/1  "phi_filtered"
  Delay1/1 -> Bus Creator/2  "p_filtered"
  Delay2/1 -> Bus Creator/3  "pdot_filtered"

== system DeployableEMF/EMF CLAWS/ACAH EMF1/Inner Loop - ACAH/[Yaw] Cmd Filter // Inv Model ==
  note: Command Filter
  note: Inverse Model
  r_cmd (rad/s) : Inport
  Vabs_kts : Inport  Port=2
  1-D Lookup Table1 : Lookup_n-D  NumberOfTableDimensions=1  BreakpointsForDimension1=EMF.VTAB  BeginIndexSearchUsingPreviousIndexResult=on  TableSource=Input port  Table=tanh([-5:5])  ExtrapMethod=Clip  InternalRulePriority=Speed  OutDataTypeStr=single  RndMeth=Simplest
      settings: InputPortMap=u0,p221
  1-D Lookup Table2 : Lookup_n-D  NumberOfTableDimensions=1  BreakpointsForDimension1=EMF.VTAB  BeginIndexSearchUsingPreviousIndexResult=on  TableSource=Input port  Table=tanh([-5:5])  ExtrapMethod=Clip  InternalRulePriority=Speed  OutDataTypeStr=single  RndMeth=Simplest
      settings: InputPortMap=u0,p221
  Bus Creator : BusCreator  Inputs=2
  Constant : Constant  Value=EMF.rTau  OutDataTypeStr=single
  Constant2 : Constant  Value=EMF.Nr  OutDataTypeStr=single
  Constant3 : Constant  Value=EMF.Nped  OutDataTypeStr=single
  Delay : Delay  DelayLength=EMF.YawDelay/framePeriod_s
  Delay1 : Delay  DelayLength=EMF.YawDelay/framePeriod_s
  Discrete-Time Integrator : DiscreteIntegrator  SampleTime=-1  OutDataTypeStr=single  ICPrevOutput=DiscIntNeverNeededParam  ICPrevScaledInput=DiscIntNeverNeededParam
  Divide : Product  Inputs=*/  OutDataTypeStr=single
  Divide1 : Product  Inputs=*/  OutDataTypeStr=single
  Product3 : Product
  Sum : Sum  Inputs=|+-
  Sum2 : Sum  Inputs=|+-
  ped_ff : Outport
  r_ideal : Outport  Port=2
  cmdFilValues : Outport  Port=3
  wires:
  [rdot_ideal] -> Delay/1  "rdot_ideal"
  Bus Creator/1 -> cmdFilValues/1
  [r_ideal] -> Delay1/1  "r_ideal"
  Divide/1 -> Discrete-Time Integrator/1, Sum2/1, [rdot_ideal]  "rdot_ideal"
  Sum2/1 -> Divide1/1
  r_cmd (rad/s)/1 -> Sum/1
  Sum/1 -> Divide/1
  Discrete-Time Integrator/1 -> Product3/2, Sum/2, r_ideal/1, [r_ideal]  "r_ideal"
  Constant/1 -> Divide/2
  Product3/1 -> Sum2/2
  Divide1/1 -> ped_ff/1
  [Vabs] -> 1-D Lookup Table1/1
  Constant2/1 -> 1-D Lookup Table1/2
  Constant3/1 -> 1-D Lookup Table2/2
  [Vabs] -> 1-D Lookup Table2/1
  1-D Lookup Table1/1 -> Product3/1
  1-D Lookup Table2/1 -> Divide1/2
  Vabs_kts/1 -> [Vabs]
  Delay/1 -> Bus Creator/1  "rdot_filtered"
  Delay1/1 -> Bus Creator/2  "r_filtered"

== system DeployableEMF/EMF CLAWS/ACAH EMF1/OnGroundController/Get ACAH Commands1 ==
  StickInputs : Inport
  Constant : Constant  Value=-1
  Constant1 : Constant
  Constant2 : Constant  Value=0
  Demux : Demux
  Gain{,1..3} (4 alike) : Gain  Gain=0
  Mux : Mux
  Saturation{,1..3} (4 alike) : Saturate  UpperLimit=1  LowerLimit=-1
  remap throttle to RPM : MATLAB Function  TreatAsAtomicUnit=on
  rotor speed : Constant  Value=mean(InitCond.TrimInputs)*2
  cmdsACAH : Outport
  throttleOmega : Outport  Port=2
  wires:
  StickInputs/1 -> Demux/1
  Demux/1 -> Saturation/1
  Demux/2 -> Saturation1/1
  Demux/3 -> Saturation2/1
  Demux/4 -> Saturation3/1
  Saturation/1 -> Gain/1
  Saturation1/1 -> Gain1/1
  Saturation3/1 -> Gain3/1
  Gain3/1 -> Mux/4
  Mux/1 -> cmdsACAH/1
  Gain1/1 -> Mux/3
  Gain/1 -> Mux/2
  Gain2/1 -> Mux/1
  rotor speed/1 -> remap throttle to RPM/5(out_max)
  Constant2/1 -> remap throttle to RPM/4(out_min)
  Constant/1 -> remap throttle to RPM/2(in_min)
  remap throttle to RPM/1(raw_out) -> throttleOmega/1  "PWM_cont"
  Saturation2/1 -> remap throttle to RPM/1(norm_in), Gain2/1
  Constant1/1 -> remap throttle to RPM/3(in_max)

== system DeployableEMF/EMF CLAWS/ACAH EMF1/OnGroundController/OL rotor speeds from throttle ==
  throttleOmega : Inport
  Gain : Gain  Gain=InitCond.Omega1_rps/mean([InitCond.Omega1_rps, InitCond.Omega2_rps])
  Gain1 : Gain  Gain=InitCond.Omega2_rps/mean([InitCond.Omega1_rps, InitCond.Omega2_rps])
  Gain2 : Gain  Gain=InitCond.Omega3_rps/mean([InitCond.Omega1_rps, InitCond.Omega2_rps])
  Gain3 : Gain  Gain=InitCond.Omega4_rps/mean([InitCond.Omega1_rps, InitCond.Omega2_rps])
  Mux2 : Mux
  Omegas_rps : Outport
  wires:
  throttleOmega/1 -> Gain3/1, Gain2/1, Gain1/1, Gain/1
  Gain/1 -> Mux2/1
  Gain1/1 -> Mux2/2
  Gain2/1 -> Mux2/3
  Gain3/1 -> Mux2/4
  Mux2/1 -> Omegas_rps/1

== system DeployableEMF/EMF CLAWS/ACAH EMF1/Remap Rotor Speeds to PWM/Rotor Speed Saturation ==
  Rotor Speeds : Inport
  Compare To Constant7 : simulink/Logic and Bit Operations/Compare To Constant  relop=<  const=AircraftModel.MinOmegaLimit(1)  OutDataTypeStr=boolean
  Compare To Constant8 : simulink/Logic and Bit Operations/Compare To Constant  relop=>  const=AircraftModel.MaxOmegaLimit(1)  OutDataTypeStr=boolean
  Logical Operator4 : Logic  Operator=OR  AllPortsSameDT=off  OutDataTypeStr=boolean
  Saturation4 : Saturate  UpperLimit=AircraftModel.MaxOmegaLimit(1)  LowerLimit=AircraftModel.MinOmegaLimit(1)
  OmegaSaturationFlags : Outport
  Saturated Rotor Speeds : Outport  Port=2
  wires:
  Saturation4/1 -> Saturated Rotor Speeds/1
  Rotor Speeds/1 -> Compare To Constant8/1, Compare To Constant7/1, Saturation4/1
  Logical Operator4/1 -> OmegaSaturationFlags/1
  Compare To Constant8/1 -> Logical Operator4/1
  Compare To Constant7/1 -> Logical Operator4/2

== matlab function DeployableEMF/command selection/throttle_norm/remap ==
  data: raw_in input; norm_out output; in_min input; in_max input; out_min input; out_max input
function norm_out = remap(raw_in,in_min,in_max,out_min,out_max)
norm_out = (raw_in - in_min) * (out_max - out_min)/(in_max-in_min) + out_min;

== matlab function DeployableEMF/command selection/yaw_norm_deadband/remap_with_deadband ==
  data: raw_in input; norm_out output; in_min input; in_max input; out_min input; out_max input; deadband input
function norm_out = remap_deadband(raw_in, in_min, in_max, out_min, out_max, deadband)
in_avg = (in_min + in_max) / 2;
out_avg = (out_min + out_max) / 2;

in_deadband_range = (in_max - in_min) * deadband / 2;
in_deadband_low = in_avg - in_deadband_range;
in_deadband_hi = in_avg + in_deadband_range;

if raw_in < in_deadband_low
    norm_out = (raw_in - in_deadband_low) .* (out_max - out_avg)./(in_deadband_low - in_min) + out_avg;
elseif raw_in > in_deadband_low && raw_in < in_deadband_hi
    norm_out = out_avg;
else
    norm_out = (raw_in - in_deadband_hi) .* (out_max - out_avg)./(in_max - in_deadband_hi) + out_avg;
end

== matlab function DeployableEMF/EMF CLAWS/ACAH EMF1/OnGroundController/Get ACAH Commands1/remap throttle to RPM ==
  data: norm_in input; raw_out output; in_min input; in_max input; out_min input; out_max input
function raw_out = remap(norm_in,in_min,in_max,out_min,out_max)
raw_out = (norm_in - in_min) * (out_max - out_min)/(in_max-in_min) + out_min;

== matlab function DeployableEMF/EMF CLAWS/ACAH EMF1/Remap Rotor Speeds to PWM/remap ==
  data: norm_in input; raw_out output; in_min input; in_max input; out_min input; out_max input
function raw_out = arrayremap(norm_in,in_min,in_max,out_min,out_max)
raw_out = norm_in*0;
for i = 1:length(norm_in)
raw_out(i) = (norm_in(i) - in_min(i)) * (out_max(i) - out_min(i))/(in_max(i)-in_min(i)) + out_min(i);
end
end

== matlab function DeployableEMF/EMF CLAWS/PWM to Linear Model Inputs/remap ==
  data: norm_in input; raw_out output; in_min input; in_max input; out_min input; out_max input
function raw_out = arrayremap(norm_in,in_min,in_max,out_min,out_max)
raw_out = norm_in*0;
for i = 1:length(norm_in)
raw_out(i) = (norm_in(i) - in_min(i)) * (out_max(i) - out_min(i))/(in_max(i)-in_min(i)) + out_min(i);
end
end

== matlab function DeployableEMF/command selection/e-stop/remap ==
  data: raw_in input; norm_out output; in_min input; in_max input; out_min input; out_max input
function norm_out = remap(raw_in,in_min,in_max,out_min,out_max)
norm_out = (raw_in - in_min) * (out_max - out_min)/(in_max-in_min) + out_min;

== matlab function DeployableEMF/command selection/mode_norm/remap ==
  data: raw_in input; norm_out output; in_min input; in_max input; out_min input; out_max input
function norm_out = remap(raw_in,in_min,in_max,out_min,out_max)
norm_out = (raw_in - in_min) * (out_max - out_min)/(in_max-in_min) + out_min;

== matlab function DeployableEMF/remap ==
  data: raw_in input; norm_out output; in_min input; in_max input; out_min input; out_max input
function norm_out = remap(raw_in,in_min,in_max,out_min,out_max)
norm_out = (raw_in - in_min) * (out_max - out_min)/(in_max-in_min) + out_min;

== matlab function DeployableEMF/command selection/pitch_norm_deadband/remap_with_deadband ==
  data: raw_in input; norm_out output; in_min input; in_max input; out_min input; out_max input; deadband input
function norm_out = remap_deadband(raw_in, in_min, in_max, out_min, out_max, deadband)
in_avg = (in_min + in_max) / 2;
out_avg = (out_min + out_max) / 2;

in_deadband_range = (in_max - in_min) * deadband / 2;
in_deadband_low = in_avg - in_deadband_range;
in_deadband_hi = in_avg + in_deadband_range;

if raw_in < in_deadband_low
    norm_out = (raw_in - in_deadband_low) .* (out_max - out_avg)./(in_deadband_low - in_min) + out_avg;
elseif raw_in > in_deadband_low && raw_in < in_deadband_hi
    norm_out = out_avg;
else
    norm_out = (raw_in - in_deadband_hi) .* (out_max - out_avg)./(in_max - in_deadband_hi) + out_avg;
end

== matlab function DeployableEMF/command selection/roll_norm_deadband/remap_with_deadband ==
  data: raw_in input; norm_out output; in_min input; in_max input; out_min input; out_max input; deadband input
function norm_out = remap_deadband(raw_in, in_min, in_max, out_min, out_max, deadband)
in_avg = (in_min + in_max) / 2;
out_avg = (out_min + out_max) / 2;

in_deadband_range = (in_max - in_min) * deadband / 2;
in_deadband_low = in_avg - in_deadband_range;
in_deadband_hi = in_avg + in_deadband_range;

if raw_in < in_deadband_low
    norm_out = (raw_in - in_deadband_low) .* (out_max - out_avg)./(in_deadband_low - in_min) + out_avg;
elseif raw_in > in_deadband_low && raw_in < in_deadband_hi
    norm_out = out_avg;
else
    norm_out = (raw_in - in_deadband_hi) .* (out_max - out_avg)./(in_max - in_deadband_hi) + out_avg;
end
